simulink model "Model"  (R2023a)
settings: Solver=FixedStepAuto  StartTime=0.0  StopTime=50  FixedStep=0.01  RelTol=1e-3
libraries: simulink x2, SignalEditorBlockLib x1
settings Model: Creator=Ahmed  LastModifiedBy=Ahmed
settings OptimizationCC: DefaultParameterBehavior=Inlined  UseDivisionForNetSlopeComputation=on  GainParamInheritBuiltInType=on  UseFloatMulNetSlope=on  InlineInvariantSignals=on  PassReuseOutputArgsAs=Individual arguments  ZeroExternalMemoryAtStartup=off  ZeroInternalMemoryAtStartup=off  NoFixptDivByZeroProtection=on  EfficientFloat2IntCast=on  LifeSpan=1  OptimizeBlockOrder=speed  DifferentSizesBufferReuse=on  EfficientTunableParamExpr=on
settings DebuggingCC: ParameterPrecisionLossMsg=none  ParameterTunabilityLossMsg=error
settings HardwareCC: ProdBitPerPointer=32  ProdBitPerSizeT=32  ProdBitPerPtrDiffT=32  ProdLargestAtomicInteger=Long  ProdLargestAtomicFloat=Double  ProdWordSize=32  ProdLongLongMode=on  ProdHWDeviceType=ARM Compatible->ARM Cortex-M
settings SFSimCC: MATLABDynamicMemAlloc=off
settings RTWCC: Description=Embedded Coder  SystemTargetFile=ert.tlc  TemplateMakefile=ert_default_tmf
settings CodeAppCC: ForceParamTrailComments=on  IgnoreCustomStorageClasses=off  OperatorAnnotations=on  SimulinkDataObjDesc=on  SFDataObjDesc=on  CustomSymbolStrGlobalVar=rt$N$M  CustomSymbolStrType=$N$M  CustomSymbolStrFcn=$N$M$F  CustomSymbolStrMacro=$N$M  InsertBlockDesc=on
settings ERTTargetCC: TargetLangStandard=C99 (ISO)  GenerateSampleERTMain=on  IncludeMdlTerminateFcn=off  CombineSignalStateStructs=on  SupportComplex=off  SupportNonInlinedSFcns=on  InlinedParameterPlacement=NonHierarchical  ERTCustomFileTemplate=example_file_process.tlc  ERTFilePackagingFormat=CompactWithDataFile

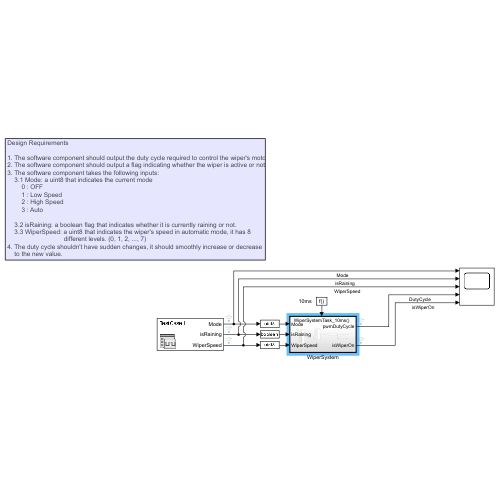
[thumbnail: Simulink's stored preview of the top-level diagram]
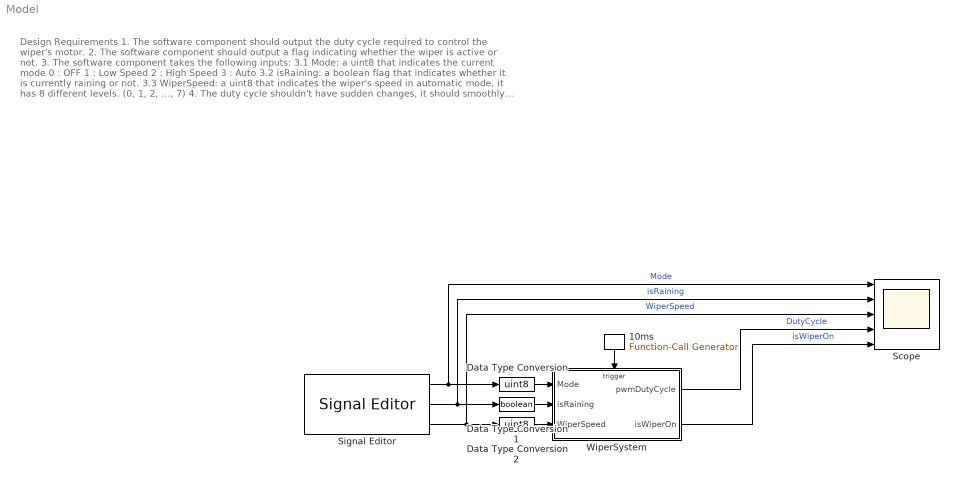
== system Model ==
  note: Design Requirements
      |
      | 1. The software component should output the duty cycle required to control the wiper's motor.
      | 2. The software component should output a flag indicating whether the wiper is active or not.
      | 3. The software component takes the following inputs:
      |     3.1 Mode: a uint8 that indicates the current mode
      |         0 : OFF
      |         1 : Low Speed
      |         2 : High Speed
      |         3 : Auto
      |
      |     3.2 isRaining: a boolean flag that indicates whether it is currently raining or not.
      |     3.3 WiperSpeed: a uint8 that indicates the wiper's speed in automatic mode, it has 8
      |                                 different levels. (0, 1, 2, ..., 7)
      | 4. The duty cycle shouldn't have sudden changes, it should smoothly increase or decrease
      |     to the new value.
  "10ms " : simulink/Ports & Subsystems/Function-Call Generator  sample_time=0.01  numberOfIterations=1  DisallowWideOutput=off
  Data Type Conversion : DataTypeConversion  OutDataTypeStr=uint8  SaturateOnIntegerOverflow=off  RndMeth=Floor
  Data Type Conversion1 : DataTypeConversion  OutDataTypeStr=boolean  SaturateOnIntegerOverflow=off  RndMeth=Floor
  Data Type Conversion2 : DataTypeConversion  OutDataTypeStr=uint8  SaturateOnIntegerOverflow=off  RndMeth=Floor
  Scope : Scope  NumInputPorts=5
  Signal Editor : SignalEditorBlockLib/Signal Editor  FileName=TestScenario.mat  ActiveScenario=TestCase1  ActiveSignal=Mode  IsBus=off  OutputBusObjectStr=Bus: BusObject  SampleTime=0  Interpolate=off  ZeroCross=off  OutputAfterFinalValue=Setting to zero  Unit=inherit  PreserveSignalName=on  ApplySigPropsToAllScenarios=on
  WiperSystem : Subsystem  TreatAsAtomicUnit=on
  wires:
  "10ms "/1 -> WiperSystem/Trigger
  Signal Editor/1 -> Scope/1, Data Type Conversion/1  "Mode"
  Signal Editor/2 -> Scope/2, Data Type Conversion1/1  "isRaining"
  Signal Editor/3 -> Scope/3, Data Type Conversion2/1  "WiperSpeed"
  Data Type Conversion/1 -> WiperSystem/1(Mode)
  Data Type Conversion1/1 -> WiperSystem/2(isRaining)
  Data Type Conversion2/1 -> WiperSystem/3(WiperSpeed)
  WiperSystem/1(pwmDutyCycle) -> Scope/4  "DutyCycle"
  WiperSystem/2(isWiperOn) -> Scope/5  "isWiperOn"

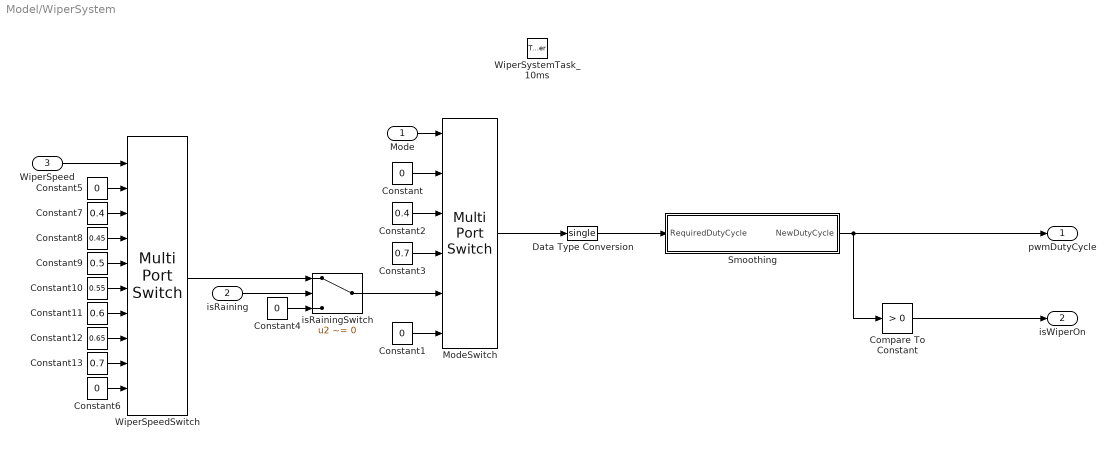
== system Model/WiperSystem ==
  Mode : Inport
  isRaining : Inport  Port=2
  WiperSpeed : Inport  Port=3
  WiperSystemTask_10ms : TriggerPort  TriggerType=function-call  VariantControl=(inherit)
  Compare To Constant : simulink/Logic and Bit Operations/Compare To Constant  relop=>  const=0  OutDataTypeStr=boolean
  Constant{,1,4..6} (5 alike) : Constant  Value=0
  Constant10 : Constant  Value=0.55
  Constant11 : Constant  Value=0.6
  Constant12 : Constant  Value=0.65
  Constant13 : Constant  Value=0.7
  Constant2 : Constant  Value=0.4
  Constant3 : Constant  Value=0.7
  Constant7 : Constant  Value=0.4
  Constant8 : Constant  Value=0.45
  Constant9 : Constant  Value=0.5
  Data Type Conversion : DataTypeConversion  OutDataTypeStr=single  SaturateOnIntegerOverflow=off  RndMeth=Floor
  ModeSwitch : MultiPortSwitch  DataPortOrder=Zero-based contiguous  Inputs=4  DataPortForDefault=Additional data port  DiagnosticForDefault=None  zeroidx=on  SaturateOnIntegerOverflow=off  InputSameDT=off
  Smoothing : Subsystem
  WiperSpeedSwitch : MultiPortSwitch  DataPortOrder=Zero-based contiguous  Inputs=8  DataPortForDefault=Additional data port  DiagnosticForDefault=None  zeroidx=on  SaturateOnIntegerOverflow=off  InputSameDT=off
  isRainingSwitch : Switch  Criteria=u2 ~= 0  SaturateOnIntegerOverflow=off  InputSameDT=off
  pwmDutyCycle : Outport
  isWiperOn : Outport  Port=2
  wires:
  Mode/1 -> ModeSwitch/1
  Constant/1 -> ModeSwitch/2
  Constant1/1 -> ModeSwitch/6
  Constant2/1 -> ModeSwitch/3
  Constant3/1 -> ModeSwitch/4
  isRaining/1 -> isRainingSwitch/2
  Constant4/1 -> isRainingSwitch/3
  Constant6/1 -> WiperSpeedSwitch/10
  WiperSpeed/1 -> WiperSpeedSwitch/1
  isRainingSwitch/1 -> ModeSwitch/5
  WiperSpeedSwitch/1 -> isRainingSwitch/1
  Constant5/1 -> WiperSpeedSwitch/2
  Constant7/1 -> WiperSpeedSwitch/3
  Constant8/1 -> WiperSpeedSwitch/4
  Constant9/1 -> WiperSpeedSwitch/5
  Constant10/1 -> WiperSpeedSwitch/6
  Constant11/1 -> WiperSpeedSwitch/7
  Constant12/1 -> WiperSpeedSwitch/8
  Constant13/1 -> WiperSpeedSwitch/9
  ModeSwitch/1 -> Data Type Conversion/1
  Smoothing/1(NewDutyCycle) -> Compare To Constant/1, pwmDutyCycle/1
  Data Type Conversion/1 -> Smoothing/1(RequiredDutyCycle)
  Compare To Constant/1 -> isWiperOn/1

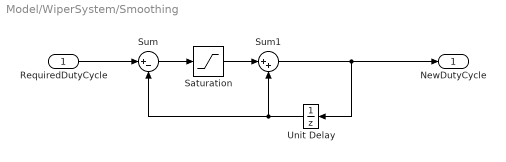
== system Model/WiperSystem/Smoothing ==
  RequiredDutyCycle : Inport
  Saturation : Saturate  UpperLimit=0.0025  LowerLimit=-0.0025
  Sum : Sum  Inputs=|+-
  Sum1 : Sum  Inputs=|++
  Unit Delay : UnitDelay  SampleTime=-1  HasFrameUpgradeWarning=on
  NewDutyCycle : Outport
  wires:
  Unit Delay/1 -> Sum/2, Sum1/2
  Sum1/1 -> NewDutyCycle/1, Unit Delay/1
  Saturation/1 -> Sum1/1
  Sum/1 -> Saturation/1
  RequiredDutyCycle/1 -> Sum/1
